simulink model "observer_only_observing"  (R2022b)
settings: Solver=VariableStepAuto  StartTime=0.0  StopTime=10.0  RelTol=1e-3
values from neighbouring files (symbols this model uses):
  K = acker(A,B, [sk sk sk])    [params.m]
  L = acker(A', C', [so so so])    [params.m]
undefined symbols (not defined in the file or in its folder): A, C
settings Model: Creator=antekgrajek  LastModifiedBy=antekgrajek

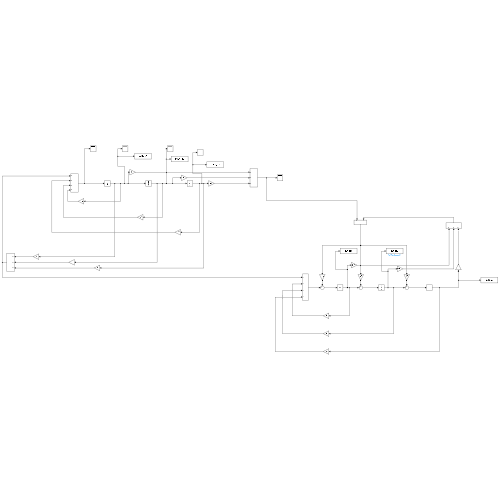
[thumbnail: Simulink's stored preview of the top-level diagram]
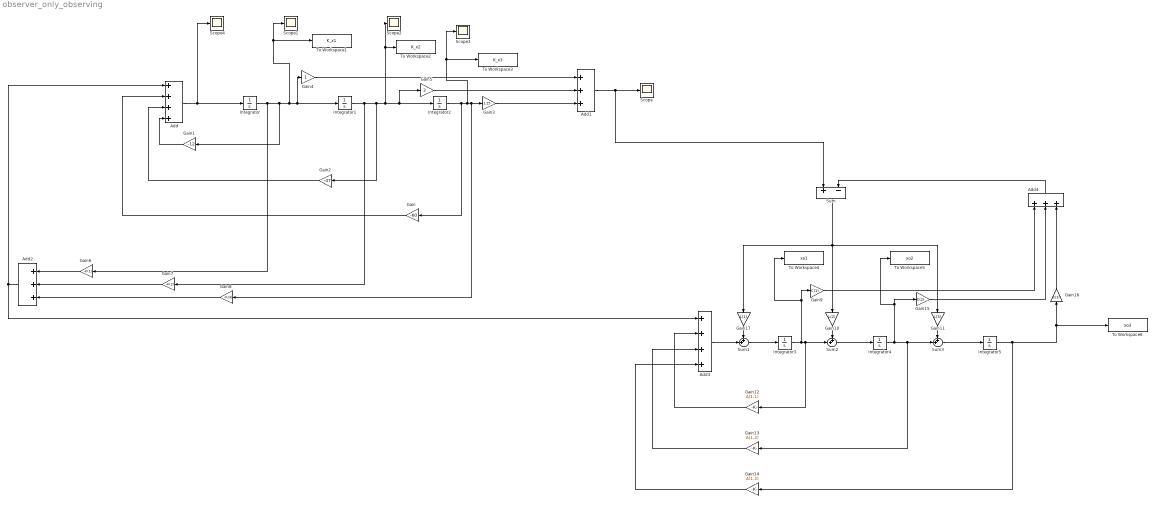
== system observer_only_observing ==
  Add : Sum  Inputs=++++
  Add1 : Sum  Inputs=+++
  Add2 : Sum  Inputs=+++
  Add3 : Sum  Inputs=++++
  Add4 : Sum  Inputs=+++
  Gain : Gain  Gain=-60
  Gain1 : Gain  Gain=-12
  Gain10 : Gain  Gain=L(2)
  Gain11 : Gain  Gain=L(3)
  Gain12 : Gain  Gain=A(1,1)
  Gain13 : Gain  Gain=A(1,2)
  Gain14 : Gain  Gain=A(1,3)
  Gain15 : Gain  Gain=C(2)
  Gain16 : Gain  Gain=C(3)
  Gain17 : Gain  Gain=L(1)
  Gain2 : Gain  Gain=-47
  Gain3 : Gain  Gain=1.25
  Gain4 : Gain
  Gain5 : Gain  Gain=3
  Gain6 : Gain  Gain=-K(1)
  Gain7 : Gain  Gain=-K(2)
  Gain8 : Gain  Gain=-K(3)
  Gain9 : Gain  Gain=C(1)
  Integrator : Integrator  InitialCondition=5
  Integrator1 : Integrator  InitialCondition=6
  Integrator2 : Integrator  InitialCondition=1
  Integrator3 : Integrator
  Integrator4 : Integrator
  Integrator5 : Integrator
  Scope{,1..4} (5 alike) : Scope
  Sum : Sum  Inputs=+-
  Sum1 : Sum  Inputs=++|
  Sum2 : Sum  Inputs=++|
  Sum3 : Sum  Inputs=++|
  To Workspace1 : ToWorkspace  VariableName=K_x1  SaveFormat=Timeseries  SampleTime=-1
  To Workspace2 : ToWorkspace  VariableName=K_x2  SaveFormat=Timeseries  SampleTime=-1
  To Workspace3 : ToWorkspace  VariableName=K_x3  SaveFormat=Timeseries  SampleTime=-1
  To Workspace4 : ToWorkspace  VariableName=xo1  SaveFormat=Timeseries  SampleTime=-1
  To Workspace5 : ToWorkspace  VariableName=xo2  SaveFormat=Timeseries  SampleTime=-1
  To Workspace6 : ToWorkspace  VariableName=xo3  SaveFormat=Timeseries  SampleTime=-1
  wires:
  Gain6/1 -> Add2/1
  Add/1 -> Scope4/1, Integrator/1
  Gain8/1 -> Add2/3
  Gain/1 -> Add/2
  Integrator1/1 -> Gain7/1, Gain2/1, To Workspace2/1, Scope2/1, Gain5/1, Integrator2/1
  Gain1/1 -> Add/4
  Integrator/1 -> Gain6/1, Gain1/1, To Workspace1/1, Scope1/1, Gain4/1, Integrator1/1
  Gain4/1 -> Add1/1
  Gain3/1 -> Add1/3
  Integrator2/1 -> Gain/1, To Workspace3/1, Scope3/1, Gain8/1, Gain3/1
  Add2/1 -> Add3/1, Add/1
  Gain7/1 -> Add2/2
  Gain2/1 -> Add/3
  Gain5/1 -> Add1/2
  Add1/1 -> Sum/1, Scope/1
  Add3/1 -> Sum1/2
  Integrator4/1 -> To Workspace5/1, Gain15/1, Gain13/1, Sum3/2
  Gain10/1 -> Sum2/1
  Gain12/1 -> Add3/2
  Integrator3/1 -> To Workspace4/1, Gain9/1, Gain12/1, Sum2/2
  Gain17/1 -> Sum1/1
  Gain11/1 -> Sum3/1
  Sum/1 -> Gain11/1, Gain10/1, Gain17/1
  Sum2/1 -> Integrator4/1
  Add4/1 -> Sum/2
  Gain16/1 -> Add4/3
  Gain14/1 -> Add3/4
  Sum1/1 -> Integrator3/1
  Gain9/1 -> Add4/1
  Gain13/1 -> Add3/3
  Gain15/1 -> Add4/2
  Integrator5/1 -> Gain14/1, To Workspace6/1, Gain16/1
  Sum3/1 -> Integrator5/1
